simulink subsystem "chute_forces"  (R2025b)
settings: Solver=VariableStepAuto  StartTime=0.0  StopTime=10.0  RelTol=1e-3
undefined symbols (not defined in the file): chute_pos_x
settings Model: Creator=finnb  LastModifiedBy=finnb

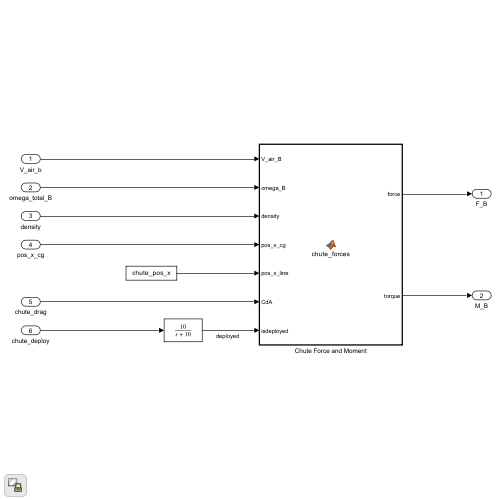
[thumbnail: Simulink's stored preview of the top-level diagram]
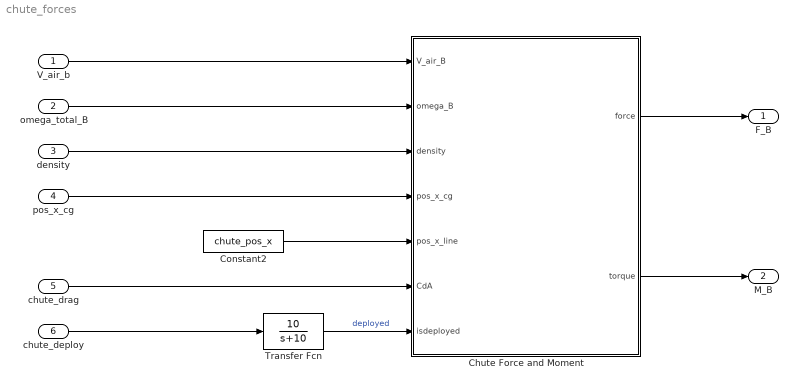
== system chute_forces ==
  V_air_b : Inport
  omega_total_B : Inport  Port=2
  "density " : Inport  Port=3
  pos_x_cg : Inport  Port=4
  chute_drag : Inport  Port=5
  chute_deploy : Inport  Port=6
  Chute Force and Moment : MATLAB Function  TreatAsAtomicUnit=on
  Constant2 : Constant  Value=chute_pos_x
  Transfer Fcn : TransferFcn  Numerator=[10]  Denominator=[1 10]
  F_B : Outport
  M_B : Outport  Port=2  VectorParamsAs1DForOutWhenUnconnected=off
  wires:
  pos_x_cg/1 -> Chute Force and Moment/4(pos_x_cg)
  Constant2/1 -> Chute Force and Moment/5(pos_x_line)
  Chute Force and Moment/2(torque) -> M_B/1
  V_air_b/1 -> Chute Force and Moment/1(V_air_B)
  omega_total_B/1 -> Chute Force and Moment/2(omega_B)
  Chute Force and Moment/1(force) -> F_B/1
  chute_drag/1 -> Chute Force and Moment/6(CdA)
  "density "/1 -> Chute Force and Moment/3(density)
  chute_deploy/1 -> Transfer Fcn/1
  Transfer Fcn/1 -> Chute Force and Moment/7(isdeployed)  "deployed"

== matlab function chute_forces/Chute Force and Moment ==
  data: force output; V_air_B input; omega_B input; density input; pos_x_cg input; pos_x_line input; CdA input; torque output; isdeployed input
function [force, torque] = chute_forces(V_air_B, omega_B, density, pos_x_cg, pos_x_line, CdA, isdeployed)
  
    % moment arm
    pos_x = (pos_x_line - pos_x_cg) * [1;0;0];

    % relative velocity
    % Vrel = V_air_B;
    V_rel = V_air_B + cross(omega_B, pos_x);

    % Line direction and damping
    V_dir = V_rel / (norm(V_rel)^1.1 + 1e-2);

    %%% Forces  
    % chute force magnitude
    F = 0.5 * density * norm(V_air_B)^2 * CdA;
    % F = min(F, 1000);

    % line force
    force = - V_dir * F * isdeployed;

    % Total torque
    torque = cross(pos_x, force);

end
